simulink model "araba_hiz_kontrol"  (Simulink 10.1)
settings: Solver=VariableStepAuto  StartTime=0.0  StopTime=stopTime  RelTol=1e-3
values from neighbouring files (symbols this model uses):
  A = 10000    [init_RC_devresi_bang_bang_kontrol.m]    (also in init_araba_hiz_kontrol.m = [0 1; 0 -b/m]; init_araba_hiz_on_off_kontrol.m = [0 1; 0 -b/m]; init_araba_hiz_pid_kontrol.m = [0 1; 0 -b/m]; init_araba_pozisyon_bang_bang_kontrol.m = [0 1; 0 -b/m])
  b = 50    [init_araba_hiz_kontrol.m]    (also in init_araba_hiz_on_off_kontrol.m; init_araba_hiz_pid_kontrol.m; init_araba_pozisyon_bang_bang_kontrol.m = 250; init_araba_pozisyon_kontrol.m)
  B = [0; 1/m]    [init_araba_hiz_kontrol.m]    (also in init_araba_hiz_on_off_kontrol.m; init_araba_hiz_pid_kontrol.m; init_araba_pozisyon_bang_bang_kontrol.m; init_araba_pozisyon_kontrol.m)
  C = 1e-4    (= 0.0001)    [init_RC_devresi.m]    (also in init_RC_devresi_bang_bang_kontrol.m; init_araba_hiz_kontrol.m = [0 1]; init_araba_hiz_on_off_kontrol.m = [0 1]; init_araba_hiz_pid_kontrol.m = [0 1])
  D = 0    [init_araba_hiz_kontrol.m]    (also in init_araba_hiz_on_off_kontrol.m; init_araba_hiz_pid_kontrol.m; init_araba_pozisyon_bang_bang_kontrol.m; init_araba_pozisyon_kontrol.m)
  Kd = 195    [init_araba_hiz_kontrol.m]    (also in init_araba_hiz_pid_kontrol.m; init_araba_pozisyon_kontrol.m = 375; init_araba_pozisyon_pid_kontrol.m = 375; init_pendulum_with_input.m = 15)
  Ki = 70    [init_araba_hiz_kontrol.m]    (also in init_araba_hiz_pid_kontrol.m; init_araba_pozisyon_kontrol.m = 0; init_araba_pozisyon_pid_kontrol.m = 0; init_pendulum_with_input.m = 10)
  Kp = 5000    [init_araba_hiz_kontrol.m]    (also in init_araba_hiz_pid_kontrol.m; init_araba_pozisyon_kontrol.m = 20; init_araba_pozisyon_pid_kontrol.m = 20; init_pendulum_with_input.m = 80)
  m = 1000    [init_araba_hiz_kontrol.m]    (also in init_araba_hiz_on_off_kontrol.m; init_araba_hiz_pid_kontrol.m; init_araba_pozisyon_bang_bang_kontrol.m; init_araba_pozisyon_kontrol.m)
  r = 5    [init_RC_devresi_bang_bang_kontrol.m]    (also in init_araba_hiz_kontrol.m = 90; init_araba_hiz_on_off_kontrol.m = 90; init_araba_hiz_pid_kontrol.m = 90; init_araba_pozisyon_bang_bang_kontrol.m = 1000)
  x10 = 0    [init_araba_hiz_kontrol.m]    (also in init_araba_hiz_on_off_kontrol.m; init_araba_hiz_pid_kontrol.m; init_araba_pozisyon_bang_bang_kontrol.m; init_araba_pozisyon_kontrol.m)
  x20 = 0    [init_araba_hiz_kontrol.m]    (also in init_araba_hiz_on_off_kontrol.m; init_araba_hiz_pid_kontrol.m; init_araba_pozisyon_bang_bang_kontrol.m; init_araba_pozisyon_kontrol.m)
libraries: simulink x1
settings Model: Creator=TULPAR  LastModifiedBy=TULPAR
settings DataIOCC: SaveFormat=Dataset  ReturnWorkspaceOutputs=on
settings OptimizationCC: LifeSpan=auto
settings DebuggingCC: UnderspecifiedInitializationDetection=Simplified  MergeDetectMultiDrivingBlocksExec=error  SFUnexpectedBacktrackingDiag=error  SFNoUnconditionalDefaultTransitionDiag=error  SFExecutionAtInitializationDiag=warning  ArithmeticOperatorsInVariantConditions=error
settings HardwareCC: ProdBitPerPointer=64  ProdBitPerSizeT=64  ProdBitPerPtrDiffT=64  ProdLargestAtomicFloat=Float  ProdIntDivRoundTo=Zero  ProdEndianess=LittleEndian  ProdWordSize=64  ProdHWDeviceType=Intel->x86-64 (Windows64)
settings ModelReferenceCC: PropagateSignalLabelsOutOfModel=on
settings SFSimCC: SimUseLocalCustomCode=on  CustomCodeUndefinedFunction=FilterOut
settings RTWCC: RTWUseLocalCustomCode=on
settings CodeAppCC: StateflowObjectComments=off
settings GRTTargetCC: TargetLangStandard=C99 (ISO)  CombineOutputUpdateFcns=on  GRTInterface=off
settings ConfigComp: CovMetricSettings=dwe  CovHtmlReporting=off  CovSaveCumulativeToWorkspaceVar=off  CovSaveSingleToWorkspaceVar=off  CovExternalEMLEnable=on

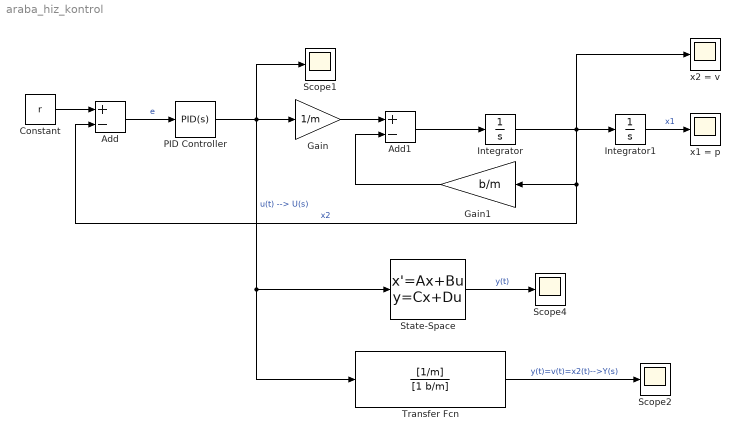
== system araba_hiz_kontrol ==
  Add : Sum  Inputs=+-
  Add1 : Sum  Inputs=+-
  Constant : Constant  Value=r
  Gain : Gain  Gain=1/m
  Gain1 : Gain  Gain=b/m
  Integrator : Integrator  InitialCondition=x20
  Integrator1 : Integrator  InitialCondition=x10
  PID Controller : simulink/Continuous/PID Controller  Controller=PID  Form=Parallel  TimeDomain=Continuous-time  UseExternalTs=off  SampleTime=-1  IntegratorMethod=Forward Euler  FilterMethod=Forward Euler  ControllerParametersSource=internal  P=Kp  I=Ki  D=Kd  UseFilter=on  N=100  TunerSelectOption=Transfer Function Based (PID Tuner App)  InitialConditionSource=internal  InitialConditionForIntegrator=0  InitialConditionForFilter=0  DifferentiatorICPrevScaledInput=0  ExternalReset=none  TrackingMode=off  Kt=1  LimitOutput=off  UpperSaturationLimit=inf  LowerSaturationLimit=-inf  LinearizeAsGain=on  AntiWindupMode=none  Kb=1  POutMin=[]  POutMax=[]  IOutMin=[]  IOutMax=[]  DOutMin=[]  DOutMax=[]  NOutMin=[]  NOutMax=[]  SumOutMin=[]  SumOutMax=[]  SaturationOutMin=[]  SaturationOutMax=[]  PParamMin=[]  PParamMax=[]  IParamMin=[]  IParamMax=[]  DParamMin=[]  DParamMax=[]  NParamMin=[]  NParamMax=[]  KbParamMin=[]  KbParamMax=[]  KtParamMin=[]  KtParamMax=[]  KbOutMin=[]  KbOutMax=[]  KtOutMin=[]  KtOutMax=[]  IntegratorOutMin=[]  IntegratorOutMax=[]  FilterOutMin=[]  FilterOutMax=[]  SumI1OutMin=[]  SumI1OutMax=[]  SumI2OutMin=[]  SumI2OutMax=[]  SumI3OutMin=[]  SumI3OutMax=[]  SumI4OutMin=[]  SumI4OutMax=[]  SumDOutMin=[]  SumDOutMax=[]  DifferentiatorOutMin=[]  DifferentiatorOutMax=[]  FilterDiffOutCoefMin=[]  FilterDiffOutCoefMax=[]  ReciprocalOutMin=[]  ReciprocalOutMax=[]  SumDenOutMin=[]  SumDenOutMax=[]  SumNumOutMin=[]  SumNumOutMax=[]  DivideOutMin=[]  DivideOutMax=[]  UdiffTsProdOutMin=[]  UdiffTsProdOutMax=[]  NTsProdOutMin=[]  NTsProdOutMax=[]  UintegralTsProdOutMin=[]  UintegralTsProdOutMax=[]  UngainTsProdOutMin=[]  UngainTsProdOutMax=[]  IntegratorContinuousStateAttributes=''  IntegratorStateMustResolveToSignalObject=off  IntegratorRTWStateStorageClass=Auto  FilterContinuousStateAttributes=''  FilterStateMustResolveToSignalObject=off  FilterRTWStateStorageClass=Auto  ParallelPVariant=InternalParameters  IdealPVariant=Disabled  IVariant=InternalParameters  DVariant=InternalParameters  IntegratorVariant=Continuous  SatVariant=Disabled  AWVariant=Passthrough  PCopyVariant=Disabled  TRVariant=Disabled  FdbkBlocksVariant=Forward  IdealPFdbkVariant=Disabled  SatFdbkVariant=Disabled  DerivativeFilterVariant=ContFilter  NVariant=InternalParameters  NCopyVariant=Disabled  FilterICVariant=InternalICsFilter  IntegratorICVariant=InternalICs  ExternalResetVariant=Disabled  TRSumVariant=Passthrough  SumFdbkVariant=Disabled  SumVariant=Sum_PID  TsampFilterVariant=InternalTs  TsampNgainVariant=Passthrough  TsampIntegralVariant=Passthrough
  Scope1 : Scope
  Scope2 : Scope
  Scope4 : Scope
  State-Space : StateSpace  A=A  B=B  C=C  D=D  InitialCondition=[x10 x20]
  Transfer Fcn : TransferFcn  Numerator=[1/m]  Denominator=[1 b/m]
  x1 = p : Scope
  x2 = v : Scope
  wires:
  Integrator1/1 -> x1 = p/1  "x1"
  Constant/1 -> Add/1
  Gain/1 -> Add1/1
  Gain1/1 -> Add1/2
  Add1/1 -> Integrator/1
  Integrator/1 -> Gain1/1, Add/2, x2 = v/1, Integrator1/1  "x2"
  Add/1 -> PID Controller/1  "e"
  PID Controller/1 -> Scope1/1, State-Space/1, Transfer Fcn/1, Gain/1  "u(t) --> U(s)"
  Transfer Fcn/1 -> Scope2/1  "y(t)=v(t)=x2(t)-->Y(s)"
  State-Space/1 -> Scope4/1  "y(t)"
